simulink model "battery_dab"  (R2025a)
settings: Solver=ode1be  StartTime=0.0  StopTime=simlength  FixedStep=ts  MaxStep=ts_sim
values from neighbouring files (symbols this model uses):
  dead_time = 0    [init_model.m]
  DThs_init = 0    [init_model.m]
  fPWM_DAB = 5e3    (= 5000)    [init_model.m]
  I_FS = Iout_dc_nom * margin_factor    (= 37.5)    [init_model.m]
  Iout_dc_nom = 30    [init_model.m]
  ki_i_dab = 18    [init_model.m]
  ki_v_dab = 45    [init_model.m]
  kp_i_dab = 2    [init_model.m]
  kp_v_dab = 8    [init_model.m]
  number_of_cells = 30    [init_model.m]
  Q = 1000    [init_model.m]
  q1Kalman = ts_dab^2    (= 4e-08)    [init_model.m]
  q2Kalman = ts_dab^1    (= 0.0002)    [init_model.m]
  q3Kalman = 0    [init_model.m]
  rKalman = 1    [init_model.m]
  Tambient = 40    [init_model.m]
  tc = ts    (= 1e-06)    [init_model.m]
  ts_dab = tPWM_DAB    (= 0.0002)    [init_model.m]
  V_FS = Vout_dc_nom * margin_factor    (= 500)    [init_model.m]
  Vout_dc_nom = 400    [init_model.m]
  weigth = 0.6/6    (= 0.1)    [init_model.m]
undefined symbols (not defined in the file or in its folder): tsample
libraries: fl_lib x79, nesl_utility x61, ee_lib x13, lithium_ion_cell_lib x1, simulink x1, single_phase_transformer_lib x1
(part 1 of 4)
settings Model: SimulationMode=accelerator  Creator=LTNBDA  LastModifiedBy=dbagn
settings SolverCC: ZeroCrossControl=EnableAll  ZeroCrossAlgorithm=Adaptive  AlgebraicLoopSolver=TrustRegion  SolverResetMethod=Robust  AutoInsertRateTranBlk=on
settings DataIOCC: LimitDataPoints=on  MaxDataPoints=1  SaveFormat=Array  SignalLoggingSaveFormat=ModelDataLogs  SaveOutput=off  SignalLogging=off  DSMLogging=off  SaveTime=off  ReturnWorkspaceOutputs=off
settings OptimizationCC: ExpressionDepthLimit=2147483647.0  InitFltsAndDblsToZero=on  EfficientMapNaN2IntZero=off  LifeSpan=inf
settings DebuggingCC: SaveWithParameterizedLinksMsg=none  UnderspecifiedInitializationDetection=Classic  MergeDetectMultiDrivingBlocksExec=none  SignalResolutionControl=TryResolveAllWithWarning  SolverPrmCheckMsg=warning  MultiTaskDSMMsg=warning  MultiTaskCondExecSysMsg=none  MultiTaskRateTransMsg=warning  FcnCallInpInsideContextMsg=warning  StateNameClashWarn=warning  SFUnexpectedBacktrackingDiag=warning  SFNoUnconditionalDefaultTransitionDiag=warning  ArithmeticOperatorsInVariantConditions=warning
settings HardwareCC: ProdBitPerLong=64.0  ProdLargestAtomicFloat=None  ProdIntDivRoundTo=Undefined  ProdEndianess=Unspecified  ProdHWDeviceType=Generic->64-bit Embedded Processor (LP64)  TargetBitPerPointer=64.0  TargetBitPerSizeT=64.0  TargetBitPerPtrDiffT=64.0  TargetLongLongMode=on  TargetIntDivRoundTo=Zero  TargetEndianess=LittleEndian  TargetWordSize=64.0  TargetHWDeviceType=MATLAB Host  ProdEqTarget=off
settings ModelReferenceCC: EnableRefExpFcnMdlSchedulingChecks=on  PropagateSignalLabelsOutOfModel=off
settings SFSimCC: SimUseLocalCustomCode=off  CustomCodeUndefinedFunction=UseInterfaceOnly
settings RTWCC: RTWUseLocalCustomCode=off  GPUComputeCapability=3.5
settings CodeAppCC: MaxIdLength=128.0  StateflowObjectComments=on
settings GRTTargetCC: TargetLangStandard=C89/C90 (ANSI)  CombineOutputUpdateFcns=off  GRTInterface=on
settings ConfigComp: CovMetricSettings=dw  CovSaveCumulativeToWorkspaceVar=on  CovSaveSingleToWorkspaceVar=on  CovExternalEMLEnable=off
settings SimscapeCC: SimscapeNormalizeSystem=off

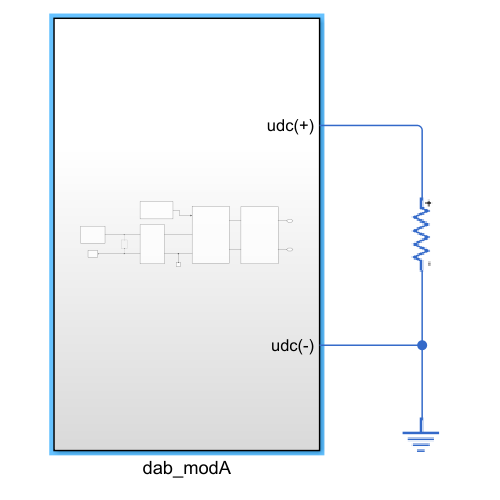
[thumbnail: Simulink's stored preview of the top-level diagram]
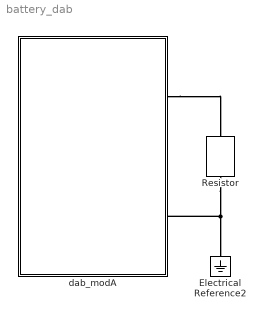
== system battery_dab ==
  Electrical Reference2 : fl_lib/Electrical/Electrical Elements/Electrical Reference
  Resistor : fl_lib/Electrical/Electrical Elements/Resistor  R=10e3 Ohm  i_specify=off  i_priority=None  i=0 A  i_nominal_specify=off  i_nominal_value=1  i_nominal_unit=A  v_specify=off  v_priority=None  v=0 V  v_nominal_specify=off  v_nominal_value=1  v_nominal_unit=V
  dab_modA : Subsystem
  connections:
  Resistor/RConn1 -- Electrical Reference2/LConn1 -- dab_modA/RConn2
  dab_modA/RConn1 -- Resistor/LConn1

== system battery_dab/dab_modA ==
  Electrical Reference : fl_lib/Electrical/Electrical Elements/Electrical Reference
  Solver Configuration : nesl_utility/Solver Configuration  PhysicalDomain=network_engine_domain  SubClassName=solver  LeftPortType=input  RightPortType=generic  Tones=[]  Harmonics=[]  SimulateNoise=off  Profile=off  UseLocalSampling=off  EnableSwitchedLinearOptims=on  FrequencyDomain=off  UseCCode=off  RelTol=0.001  AbsTol=0.001  MinStep=1e-09  ToWorkspace=off  RevertToSquareIcSolve=off  NumHomotopyIterations=100  PhasorMode=off  PhasorModeNumHarmonics=1  ConsistencySolver=NEWTON_FTOL  IndexReductionMethod=DerivativeReplacement  DoDC=on  ResidualTolerance=1e-09  ConsistencyTolSource=GLOBAL  ConsistencyAbsTol=0.001  ConsistencyRelTol=0.001  ConsistencyTolFactor=0.001  UseLocalSolver=on  LocalSolverChoice=NE_BACKWARD_EULER_ADVANCER  ResolveIndetEquations=on  FunctionEvalNumThread=1  LocalSolverSampleTime=ts  DoFixedCost=on  MaxNonlinIter=3  MaxModeIter=2  ComputeImpulses=off  ImpulseIterations=2  LinearAlgebra=auto  LinearAlgebraNumThread=0  EquationFormulation=NE_TIME_EF  DelaysMemoryBudget=1024  AutomaticFiltering=on  FilteringTimeConstant=0.001  PartitionStorageMethod=AS_NEEDED  PartitionMemoryBudget=1024  PartitionMethod=ROBUST  MultibodyUseLocalSolver=off  MultibodyLocalSolverChoice=ODE1  MultibodyLocalSolverSampleTime=0.001
  Voltage Source : ee_lib/Sources/Voltage Source  Commented=on  dc_voltage=90 V  ac_voltage=0 V  ac_shift=0 rad  ac_frequency=60 Hz  noise_mode=ee.enum.sources.noise.Disabled  PSD=0 V^2/Hz  sample_time=1e-3 s  repeatability=ee.enum.sources.repeatability.NotRepeatable  user_seed=0  auto_seed=3499211588  i_specify=off  i_priority=None  i=0 A  i_nominal_specify=off  i_nominal_value=1  i_nominal_unit=A  v_specify=off  v_priority=None  v=0 V  v_nominal_specify=off  v_nominal_value=1  v_nominal_unit=V
  battery_system : Subsystem
  dab : Subsystem
  dab_ctrl : Subsystem
  single_phase_ui_measure1 : Subsystem
  ui_measure : Subsystem
  udc(+) : PMIOPort  Side=Right
  udc(-) : PMIOPort  Port=2  Side=Right
  wires:
  dab_ctrl/1(gate_commands) -> dab/1(gate_commands)
  connections:
  dab/RConn1 -- ui_measure/LConn1
  dab/RConn2 -- ui_measure/LConn2
  udc(+)/RConn1 -- ui_measure/RConn1
  udc(-)/RConn1 -- ui_measure/RConn2
  dab/LConn2 -- single_phase_ui_measure1/RConn2 -- Electrical Reference/LConn1
  battery_system/RConn1 -- Voltage Source/LConn1 -- single_phase_ui_measure1/LConn1
  single_phase_ui_measure1/RConn1 -- dab/LConn1
  single_phase_ui_measure1/LConn2 -- Solver Configuration/RConn1 -- Voltage Source/RConn1

== system battery_dab/dab_modA/battery_system ==
  Electrical Reference1 : fl_lib/Electrical/Electrical Elements/Electrical Reference
  LithiumIonBattery : Subsystem
  Uout+ : PMIOPort  Side=Right
  connections:
  LithiumIonBattery/RConn2 -- Electrical Reference1/LConn1
  LithiumIonBattery/RConn1 -- Uout+/RConn1

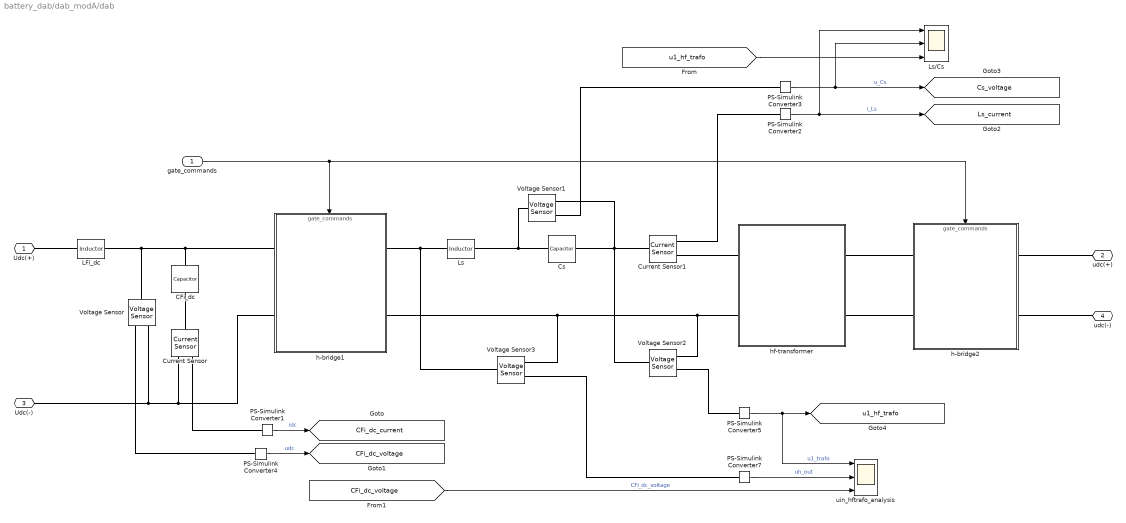
== system battery_dab/dab_modA/dab ==
  gate_commands : Inport
  CFi_dc : fl_lib/Electrical/Electrical Elements/Capacitor  c=CFi_dc F  r=RCFi_dc_internal Ohm  g=0 1/Ohm  i_specify=off  i_priority=None  i=0 A  i_nominal_specify=off  i_nominal_value=1  i_nominal_unit=A  v_specify=off  v_priority=None  v=0 V  v_nominal_specify=off  v_nominal_value=1  v_nominal_unit=V  vc_specify=off  vc_priority=High  vc=0 V  vc_nominal_specify=off  vc_nominal_value=1  vc_nominal_unit=V
  Cs : fl_lib/Electrical/Electrical Elements/Capacitor  c=Cs1 F  r=1e-6 Ohm  g=0 1/Ohm  i_specify=off  i_priority=None  i=0 A  i_nominal_specify=off  i_nominal_value=1  i_nominal_unit=A  v_specify=off  v_priority=None  v=0 V  v_nominal_specify=off  v_nominal_value=1  v_nominal_unit=V  vc_specify=off  vc_priority=High  vc=0 V  vc_nominal_specify=off  vc_nominal_value=1  vc_nominal_unit=V
  Current Sensor : fl_lib/Electrical/Electrical Sensors/Current Sensor
  Current Sensor1 : fl_lib/Electrical/Electrical Sensors/Current Sensor
  LFi_dc : fl_lib/Electrical/Electrical Elements/Inductor  l=10e-6 H  r=0 Ohm  g=1e-9 1/Ohm  i_specify=off  i_priority=None  i=0 A  i_nominal_specify=off  i_nominal_value=1  i_nominal_unit=A  v_specify=off  v_priority=None  v=0 V  v_nominal_specify=off  v_nominal_value=1  v_nominal_unit=V  i_L_specify=off  i_L_priority=High  i_L=0 A  i_L_nominal_specify=off  i_L_nominal_value=1  i_L_nominal_unit=A
  Ls : fl_lib/Electrical/Electrical Elements/Inductor  l=Ls1 H  r=0 Ohm  g=1e-9 1/Ohm  i_specify=off  i_priority=None  i=0 A  i_nominal_specify=off  i_nominal_value=1  i_nominal_unit=A  v_specify=off  v_priority=None  v=0 V  v_nominal_specify=off  v_nominal_value=1  v_nominal_unit=V  i_L_specify=off  i_L_priority=High  i_L=0 A  i_L_nominal_specify=off  i_L_nominal_value=1  i_L_nominal_unit=A
  Ls/Cs : Scope  NumInputPorts=3
      settings: SampleTime=tc  ActiveDisplayYMinimum=1.6E-10  ActiveDisplayYMaximum=3.6E-10
  PS-Simulink Converter1 : nesl_utility/PS-Simulink Converter  PhysicalDomain=network_engine_domain  SubClassName=ps_output  LeftPortType=input  RightPortType=output  PseudoPeriodic=off  Frequencies=[]  VectorFormat=1-D array  Unit=A  AffineConversion=on
  PS-Simulink Converter2 : nesl_utility/PS-Simulink Converter  PhysicalDomain=network_engine_domain  SubClassName=ps_output  LeftPortType=input  RightPortType=output  PseudoPeriodic=off  Frequencies=[]  VectorFormat=1-D array  Unit=A  AffineConversion=on
  PS-Simulink Converter{3..5,7} (4 alike) : nesl_utility/PS-Simulink Converter  PhysicalDomain=network_engine_domain  SubClassName=ps_output  LeftPortType=input  RightPortType=output  PseudoPeriodic=off  Frequencies=[]  VectorFormat=1-D array  Unit=V  AffineConversion=on
  Voltage Sensor{,1..3} (4 alike) : fl_lib/Electrical/Electrical Sensors/Voltage Sensor
  h-bridge1 : Subsystem
      settings: PortSchema="{\"entries\":[{\"content\":{\"sides\":[{\"content\":{\"connectorIds\":[\"LConn1\",\"LConn2\"]},\"type\":\"ConnectorPlacement.EquallySpacedRectSide\",\"uuid\":\"c872503a-61af-4937-bdf2-4de4f8645573\"},{\"content\":{\"connectorIds\":[\"RConn1\",\"RConn2\"],\"side\":\"RIGHT\"},\"type\":\"ConnectorPlacement.EquallySpacedRectSide\",\"uuid\":\"3b83f060-86a2-4569-84b5-d9f7c0485347\"},{\"content\":{\"connectorIds\":[\"In1\"],\"side\":\"TOP\"},\"type\":\"ConnectorPlacement.EquallySpacedRectSide\",\"uuid\":\"bf191d46-ce71-4d15-9dd0-24cc57253577\"}]},\"type\":\"ConnectorPlacement.EquallySpacedConnector\",\"uuid\":\"1b28ceee-25d0-45ae-a3c4-c2563f0d63ba\"}],\"packageUris\":[\"http://schema.mathworks.com/mf0/Connector/R2020b\"],\"version\":\"1.0\"}"
  h-bridge2 : Subsystem
      settings: PortSchema="{\"entries\":[{\"content\":{\"sides\":[{\"content\":{\"connectorIds\":[\"LConn1\",\"LConn2\"]},\"type\":\"ConnectorPlacement.EquallySpacedRectSide\",\"uuid\":\"c872503a-61af-4937-bdf2-4de4f8645573\"},{\"content\":{\"connectorIds\":[\"RConn1\",\"RConn2\"],\"side\":\"RIGHT\"},\"type\":\"ConnectorPlacement.EquallySpacedRectSide\",\"uuid\":\"3b83f060-86a2-4569-84b5-d9f7c0485347\"},{\"content\":{\"connectorIds\":[\"In1\"],\"side\":\"TOP\"},\"type\":\"ConnectorPlacement.EquallySpacedRectSide\",\"uuid\":\"bf191d46-ce71-4d15-9dd0-24cc57253577\"}]},\"type\":\"ConnectorPlacement.EquallySpacedConnector\",\"uuid\":\"1b28ceee-25d0-45ae-a3c4-c2563f0d63ba\"}],\"packageUris\":[\"http://schema.mathworks.com/mf0/Connector/R2020b\"],\"version\":\"1.0\"}"
  hf-transformer : Subsystem
  uin_hftrafo_analysis : Scope  NumInputPorts=3
      settings: SampleTime=tc  ActiveDisplayYMinimum=-95.8679  ActiveDisplayYMaximum=95.88555
  Udc(+) : PMIOPort  Side=Left
  udc(+) : PMIOPort  Port=2  Side=Right
  Udc(-) : PMIOPort  Port=3  Side=Left
  udc(-) : PMIOPort  Port=4  Side=Right
  tag scope: CFi_dc_current=global, CFi_dc_voltage=global, Cs_voltage=global, Ls_current=global, u1_hf_trafo=global
  wires:
  gate_commands/1 -> h-bridge2/1(gate_commands), h-bridge1/1(gate_commands)
  PS-Simulink Converter1/1 -> [CFi_dc_current]  "idc"
  PS-Simulink Converter4/1 -> [CFi_dc_voltage]  "udc"
  PS-Simulink Converter2/1 -> Ls/Cs/1, [Ls_current]  "i_Ls"
  PS-Simulink Converter3/1 -> Ls/Cs/2, [Cs_voltage]  "u_Cs"
  PS-Simulink Converter5/1 -> uin_hftrafo_analysis/1, [u1_hf_trafo]  "u1_trafo"
  [u1_hf_trafo] -> Ls/Cs/3
  PS-Simulink Converter7/1 -> uin_hftrafo_analysis/2  "uh_out"
  [CFi_dc_voltage] -> uin_hftrafo_analysis/3  "CFi_dc_voltage"
  connections:
  hf-transformer/LConn2 -- Voltage Sensor2/RConn2 -- Voltage Sensor3/RConn2 -- h-bridge1/LConn2
  h-bridge1/RConn1 -- CFi_dc/LConn1 -- LFi_dc/RConn1 -- Voltage Sensor/LConn1
  h-bridge1/RConn2 -- Current Sensor/RConn2 -- Udc(-)/RConn1 -- Voltage Sensor/RConn2
  LFi_dc/LConn1 -- Udc(+)/RConn1
  Current Sensor/LConn1 -- CFi_dc/RConn1
  Current Sensor/RConn1 -- PS-Simulink Converter1/LConn1
  PS-Simulink Converter4/LConn1 -- Voltage Sensor/RConn1
  h-bridge1/LConn1 -- Voltage Sensor3/LConn1 -- Ls/LConn1
  Current Sensor1/RConn2 -- hf-transformer/LConn1
  PS-Simulink Converter2/LConn1 -- Current Sensor1/RConn1
  Voltage Sensor1/RConn1 -- PS-Simulink Converter3/LConn1
  Voltage Sensor2/RConn1 -- PS-Simulink Converter5/LConn1
  Voltage Sensor1/RConn2 -- Cs/RConn1 -- Current Sensor1/LConn1 -- Voltage Sensor2/LConn1
  Ls/RConn1 -- Voltage Sensor1/LConn1 -- Cs/LConn1
  Voltage Sensor3/RConn1 -- PS-Simulink Converter7/LConn1
  hf-transformer/RConn1 -- h-bridge2/LConn1
  hf-transformer/RConn2 -- h-bridge2/LConn2
  udc(+)/RConn1 -- h-bridge2/RConn1
  udc(-)/RConn1 -- h-bridge2/RConn2

== system battery_dab/dab_modA/dab_ctrl ==
  Bus Creator : BusCreator  Inputs=8
  modulator1 : Subsystem
  references : Subsystem
  sampling_i_filter1 : Subsystem
  sampling_v_filter1 : Subsystem
  sampling_v_filter2 : Subsystem
  vi ctrl : Subsystem
  gate_commands : Outport
  wires:
  [dab_voltage_output_modA] -> sampling_v_filter1/1(in)
  [dab_current_output_modA] -> sampling_i_filter1/1(in)
  vi ctrl/1(phase_displacement) -> modulator1/1(phase_displacement)
  sampling_i_filter1/1(out_pu) -> vi ctrl/1(iout)
  sampling_v_filter1/1(out_pu) -> vi ctrl/2(vout)
  sampling_v_filter2/1(out_pu) -> vi ctrl/3(vout_ref)
  references/1(vout_ref) -> sampling_v_filter2/1(in)
  Bus Creator/1 -> gate_commands/1
  modulator1/1(gate_Q1) -> Bus Creator/1
  modulator1/2(gate_Q2) -> Bus Creator/2
  modulator1/3(gate_Q3) -> Bus Creator/3
  modulator1/4(gate_Q4) -> Bus Creator/4
  modulator1/5(gate_Q5) -> Bus Creator/5
  modulator1/6(gate_Q6) -> Bus Creator/6
  modulator1/7(gate_Q7) -> Bus Creator/7
  modulator1/8(gate_Q8) -> Bus Creator/8

== system battery_dab/dab_modA/single_phase_ui_measure1 ==
  Bus Creator : BusCreator  Inputs=2
  Current Sensor : fl_lib/Electrical/Electrical Sensors/Current Sensor
  Selector : Selector  InputPortWidth=2  IndexOptions=Index vector (dialog)  Indices=2  OutputSizes=1
  Selector1 : Selector  InputPortWidth=2  IndexOptions=Index vector (dialog)  Indices=1  OutputSizes=1
  Voltage Sensor : fl_lib/Electrical/Electrical Sensors/Voltage Sensor
  input : Scope  NumInputPorts=2
      settings: SampleTime=tc  ActiveDisplayYMinimum=-46.75689  ActiveDisplayYMaximum=366.30967  DataLoggingVariableName=ScopeData2
  iph : nesl_utility/PS-Simulink Converter  PhysicalDomain=network_engine_domain  SubClassName=ps_output  LeftPortType=input  RightPortType=output  PseudoPeriodic=off  Frequencies=[]  VectorFormat=1-D array  Unit=A  AffineConversion=off
  uph : nesl_utility/PS-Simulink Converter  PhysicalDomain=network_engine_domain  SubClassName=ps_output  LeftPortType=input  RightPortType=output  PseudoPeriodic=off  Frequencies=[]  VectorFormat=1-D array  Unit=V  AffineConversion=off
  Udc(+) : PMIOPort  Side=Left
  udc(+) : PMIOPort  Port=2  Side=Right
  Udc(-) : PMIOPort  Port=3  Side=Left
  udc(-) : PMIOPort  Port=4  Side=Right
  tag scope: current_battery=global, voltage_battery=global
  wires:
  Bus Creator/1 -> Selector/1, Selector1/1  "ui_data"
  iph/1 -> Bus Creator/1  "iph"
  uph/1 -> Bus Creator/2  "uph"
  Selector1/1 -> [current_battery], input/1  "current_battery"
  Selector/1 -> input/2, [voltage_battery]  "voltage_battery"
  connections:
  iph/LConn1 -- Current Sensor/RConn1
  Voltage Sensor/LConn1 -- Current Sensor/LConn1 -- Udc(+)/RConn1
  Current Sensor/RConn2 -- udc(+)/RConn1
  Voltage Sensor/RConn1 -- uph/LConn1
  Voltage Sensor/RConn2 -- Udc(-)/RConn1 -- udc(-)/RConn1

== system battery_dab/dab_modA/ui_measure ==
  Bus Creator : BusCreator  Inputs=2
  Current Sensor : fl_lib/Electrical/Electrical Sensors/Current Sensor
  Selector : Selector  InputPortWidth=2  IndexOptions=Index vector (dialog)  Indices=2  OutputSizes=1
  Selector1 : Selector  InputPortWidth=2  IndexOptions=Index vector (dialog)  Indices=1  OutputSizes=1
  Voltage Sensor : fl_lib/Electrical/Electrical Sensors/Voltage Sensor
  idc/udc dab modA : Scope  NumInputPorts=2
      settings: SampleTime=tc  ActiveDisplayYMinimum=4E-31  ActiveDisplayYMaximum=1.7E-30  DataLoggingVariableName=ScopeData2
  iph : nesl_utility/PS-Simulink Converter  PhysicalDomain=network_engine_domain  SubClassName=ps_output  LeftPortType=input  RightPortType=output  PseudoPeriodic=off  Frequencies=[]  VectorFormat=1-D array  Unit=A  AffineConversion=off
  uph : nesl_utility/PS-Simulink Converter  PhysicalDomain=network_engine_domain  SubClassName=ps_output  LeftPortType=input  RightPortType=output  PseudoPeriodic=off  Frequencies=[]  VectorFormat=1-D array  Unit=V  AffineConversion=off
  Udc(+) : PMIOPort  Side=Left
  udc(+) : PMIOPort  Port=2  Side=Right
  Udc(-) : PMIOPort  Port=3  Side=Left
  udc(-) : PMIOPort  Port=4  Side=Right
  tag scope: dab_current_output_modA=global, dab_voltage_output_modA=global
  wires:
  [dab_current_output_modA] -> idc/udc dab modA/1  "dab_current_output_modA"
  [dab_voltage_output_modA] -> idc/udc dab modA/2  "zvs_voltage_output_modA"
  Selector1/1 -> [dab_current_output_modA]
  Selector/1 -> [dab_voltage_output_modA]
  Bus Creator/1 -> Selector/1, Selector1/1  "ui_data"
  iph/1 -> Bus Creator/1  "iph"
  uph/1 -> Bus Creator/2  "uph"
  connections:
  iph/LConn1 -- Current Sensor/RConn1
  Voltage Sensor/LConn1 -- Current Sensor/LConn1 -- Udc(+)/RConn1
  Current Sensor/RConn2 -- udc(+)/RConn1
  Voltage Sensor/RConn1 -- uph/LConn1
  Voltage Sensor/RConn2 -- Udc(-)/RConn1 -- udc(-)/RConn1

== system battery_dab/dab_modA/battery_system/LithiumIonBattery ==
  Current Sensor : fl_lib/Electrical/Electrical Sensors/Current Sensor
  Electrical Reference1 : fl_lib/Electrical/Electrical Elements/Electrical Reference
  PS-Simulink Converter4 : nesl_utility/PS-Simulink Converter  PhysicalDomain=network_engine_domain  SubClassName=ps_output  LeftPortType=input  RightPortType=output  PseudoPeriodic=off  Frequencies=[]  VectorFormat=1-D array  Unit=1  AffineConversion=off
  PS-Simulink Converter5 : nesl_utility/PS-Simulink Converter  PhysicalDomain=network_engine_domain  SubClassName=ps_output  LeftPortType=input  RightPortType=output  PseudoPeriodic=off  Frequencies=[]  VectorFormat=1-D array  Unit=V  AffineConversion=on
  SOC_estimator : Subsystem
  To Workspace1 : ToWorkspace  VariableName=idc_battery_sim  SampleTime=tc
      settings: MaxDataPoints=Nc
  To Workspace2 : ToWorkspace  VariableName=udc_battery_sim  SampleTime=tc
      settings: MaxDataPoints=Nc
  Unit Delay5 : UnitDelay  SampleTime=ts_dab  HasFrameUpgradeWarning=on
  Voltage Sensor : fl_lib/Electrical/Electrical Sensors/Voltage Sensor
  ibat/vdc : Scope  NumInputPorts=2
      settings: SampleTime=tc  ActiveDisplayYMinimum=102.29193  ActiveDisplayYMaximum=106.82602  DataLoggingVariableName=ScopeData6
  lithium ion cell analytical ocv : Subsystem
  Uout+ : PMIOPort  Side=Right
  Uout- : PMIOPort  Port=2  Side=Right
  wires:
  PS-Simulink Converter5/1 -> Unit Delay5/1
  PS-Simulink Converter4/1 -> To Workspace1/1, ibat/vdc/1  "i batt"
  Unit Delay5/1 -> To Workspace2/1, [vdc]
  [vdc] -> ibat/vdc/2  "vdc"
  connections:
  Current Sensor/RConn1 -- PS-Simulink Converter4/LConn1
  Uout+/RConn1 -- Current Sensor/RConn2 -- Voltage Sensor/LConn1
  Voltage Sensor/RConn1 -- PS-Simulink Converter5/LConn1
  Voltage Sensor/RConn2 -- Electrical Reference1/LConn1 -- lithium ion cell analytical ocv/RConn2 -- Uout-/RConn1
  lithium ion cell analytical ocv/RConn1 -- Current Sensor/LConn1

== system battery_dab/dab_modA/dab/h-bridge1 ==
  gate_commands : Inport
  Current Sensor : fl_lib/Electrical/Electrical Sensors/Current Sensor
  PS-Simulink Converter1 : nesl_utility/PS-Simulink Converter  PhysicalDomain=network_engine_domain  SubClassName=ps_output  LeftPortType=input  RightPortType=output  PseudoPeriodic=off  Frequencies=[]  VectorFormat=1-D array  Unit=A  AffineConversion=on
  h-bridge_thermal : Subsystem  Commented=on
  h-ideal : Subsystem  Commented=on
  h-mosfet : Subsystem
  uac_1(+) : PMIOPort  Side=Left
  uac_1(-) : PMIOPort  Port=2  Side=Left
  Udc(+) : PMIOPort  Port=3  Side=Right
  Udc(-) : PMIOPort  Port=4  Side=Right
  tag scope: dc_bus_terminal_current_inverter=global
  wires:
  gate_commands/1 -> h-mosfet/1(gate_commands)
  PS-Simulink Converter1/1 -> [dc_bus_terminal_current_inverter]  "idc"
  connections:
  h-mosfet/LConn1 -- uac_1(+)/RConn1
  h-mosfet/LConn2 -- uac_1(-)/RConn1
  h-mosfet/RConn2 -- Udc(-)/RConn1
  Current Sensor/LConn1 -- Udc(+)/RConn1
  h-mosfet/RConn1 -- Current Sensor/RConn2
  PS-Simulink Converter1/LConn1 -- Current Sensor/RConn1

== system battery_dab/dab_modA/dab/h-bridge2 ==
  gate_commands : Inport
  CFu_dc : fl_lib/Electrical/Electrical Elements/Capacitor  c=CFu_dc F  r=RCFu_dc_internal Ohm  g=0 1/Ohm  i_specify=off  i_priority=None  i=0 A  i_nominal_specify=off  i_nominal_value=1  i_nominal_unit=A  v_specify=off  v_priority=None  v=0 V  v_nominal_specify=off  v_nominal_value=1  v_nominal_unit=V  vc_specify=off  vc_priority=High  vc=0 V  vc_nominal_specify=off  vc_nominal_value=1  vc_nominal_unit=V
  Current Sensor : fl_lib/Electrical/Electrical Sensors/Current Sensor
  Current Sensor2 : fl_lib/Electrical/Electrical Sensors/Current Sensor
  PS-Simulink Converter1 : nesl_utility/PS-Simulink Converter  PhysicalDomain=network_engine_domain  SubClassName=ps_output  LeftPortType=input  RightPortType=output  PseudoPeriodic=off  Frequencies=[]  VectorFormat=1-D array  Unit=A  AffineConversion=on
  PS-Simulink Converter6 : nesl_utility/PS-Simulink Converter  PhysicalDomain=network_engine_domain  SubClassName=ps_output  LeftPortType=input  RightPortType=output  PseudoPeriodic=off  Frequencies=[]  VectorFormat=1-D array  Unit=A  AffineConversion=on
  PS-Simulink Converter8 : nesl_utility/PS-Simulink Converter  PhysicalDomain=network_engine_domain  SubClassName=ps_output  LeftPortType=input  RightPortType=output  PseudoPeriodic=off  Frequencies=[]  VectorFormat=1-D array  Unit=V  AffineConversion=on
  Voltage Sensor4 : fl_lib/Electrical/Electrical Sensors/Voltage Sensor
  h-mosfet : Subsystem
  uac_1(+) : PMIOPort  Side=Left
  uac_1(-) : PMIOPort  Port=2  Side=Left
  udc(+) : PMIOPort  Port=3  Side=Right
  udc(-) : PMIOPort  Port=4  Side=Right
  tag scope: CFu_dc_current=global, CFu_dc_voltage=global
  wires:
  gate_commands/1 -> h-mosfet/1(gate_commands)
  PS-Simulink Converter6/1 -> [CFu_dc_current]  "i_Ls"
  PS-Simulink Converter8/1 -> [CFu_dc_voltage]  "CFu_dc_voltage"
  connections:
  h-mosfet/RConn1 -- Current Sensor/LConn1 -- CFu_dc/LConn1
  Voltage Sensor4/LConn1 -- udc(+)/RConn1 -- Current Sensor/RConn2
  h-mosfet/RConn2 -- Current Sensor2/RConn2 -- udc(-)/RConn1 -- Voltage Sensor4/RConn2
  h-mosfet/LConn2 -- uac_1(-)/RConn1
  h-mosfet/LConn1 -- uac_1(+)/RConn1
  Voltage Sensor4/RConn1 -- PS-Simulink Converter8/LConn1
  PS-Simulink Converter6/LConn1 -- Current Sensor2/RConn1
  CFu_dc/RConn1 -- Current Sensor2/LConn1
  Current Sensor/RConn1 -- PS-Simulink Converter1/LConn1

== system battery_dab/dab_modA/dab/hf-transformer ==
  Current Sensor1 : fl_lib/Electrical/Electrical Sensors/Current Sensor
  PS-Simulink Converter2 : nesl_utility/PS-Simulink Converter  PhysicalDomain=network_engine_domain  SubClassName=ps_output  LeftPortType=input  RightPortType=output  PseudoPeriodic=off  Frequencies=[]  VectorFormat=1-D array  Unit=A  AffineConversion=on
  hf_trafo_center_tap_ss : Subsystem
  uac_1(+) : PMIOPort  Side=Left
  uac_2(+) : PMIOPort  Port=2  Side=Right
  uac_1(-) : PMIOPort  Port=3  Side=Left
  uac_2(-) : PMIOPort  Port=4  Side=Right
  connections:
  Current Sensor1/RConn2 -- uac_2(+)/RConn1
  PS-Simulink Converter2/LConn1 -- Current Sensor1/RConn1
  hf_trafo_center_tap_ss/LConn1 -- uac_1(+)/RConn1
  hf_trafo_center_tap_ss/RConn1 -- Current Sensor1/LConn1
  hf_trafo_center_tap_ss/LConn2 -- uac_1(-)/RConn1
  hf_trafo_center_tap_ss/RConn2 -- uac_2(-)/RConn1

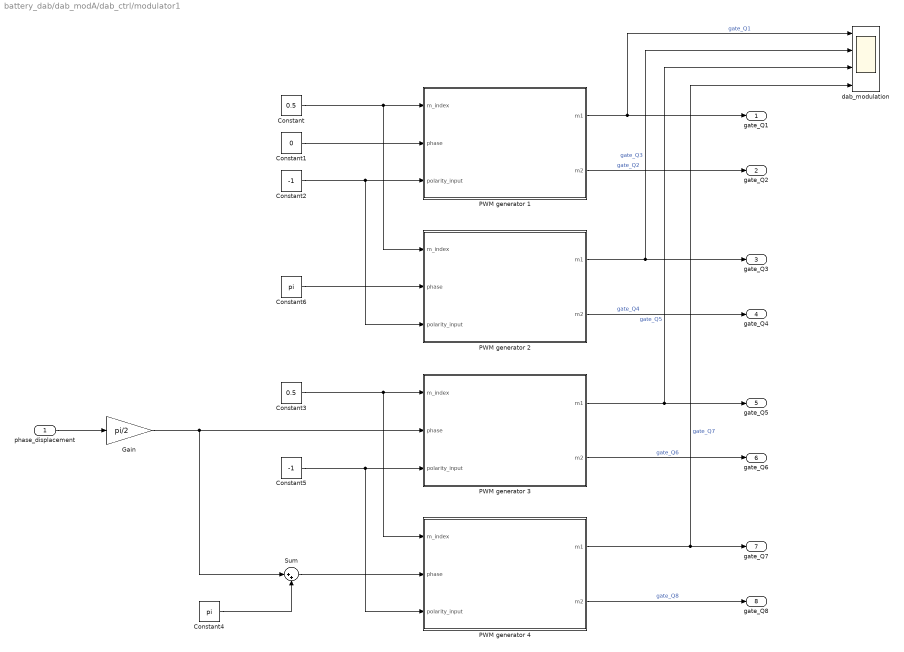
== system battery_dab/dab_modA/dab_ctrl/modulator1 ==
  phase_displacement : Inport
  Constant : Constant  Value=0.5
  Constant1 : Constant  Value=0
  Constant2 : Constant  Value=-1
  Constant3 : Constant  Value=0.5
  Constant4 : Constant  Value=pi
  Constant5 : Constant  Value=-1
  Constant6 : Constant  Value=pi
  Gain : Gain  Gain=pi/2  OutDataTypeStr=double
  PWM generator 1 : Subsystem  mask{f=fPWM_DAB, m_up=1, m_low=0, dead_time=dead_time, pos_cmd_gate=15, neg_cmd_gate=-10, polarity=1}
      mask prompts: f "Frequency (Hz)"; m_up "Max Input Modulation Value"; m_low "Min Input Modulation Value"; dead_time "Dead Time (s)"; pos_cmd_gate "Positive Gate Voltage (V)"; neg_cmd_gate "Negative Gate Voltage (V)"; polarity "Polarity (pu)"
  PWM generator 2 : Subsystem  mask{f=fPWM_DAB, m_up=1, m_low=0, dead_time=dead_time, pos_cmd_gate=15, neg_cmd_gate=-10, polarity=1}
      mask prompts: f "Frequency (Hz)"; m_up "Max Input Modulation Value"; m_low "Min Input Modulation Value"; dead_time "Dead Time (s)"; pos_cmd_gate "Positive Gate Voltage (V)"; neg_cmd_gate "Negative Gate Voltage (V)"; polarity "Polarity (pu)"
  PWM generator 3 : Subsystem  mask{f=fPWM_DAB, m_up=1, m_low=0, dead_time=dead_time, pos_cmd_gate=15, neg_cmd_gate=-10, polarity=1}
      mask prompts: f "Frequency (Hz)"; m_up "Max Input Modulation Value"; m_low "Min Input Modulation Value"; dead_time "Dead Time (s)"; pos_cmd_gate "Positive Gate Voltage (V)"; neg_cmd_gate "Negative Gate Voltage (V)"; polarity "Polarity (pu)"
  PWM generator 4 : Subsystem  mask{f=fPWM_DAB, m_up=1, m_low=0, dead_time=dead_time, pos_cmd_gate=15, neg_cmd_gate=-10, polarity=1}
      mask prompts: f "Frequency (Hz)"; m_up "Max Input Modulation Value"; m_low "Min Input Modulation Value"; dead_time "Dead Time (s)"; pos_cmd_gate "Positive Gate Voltage (V)"; neg_cmd_gate "Negative Gate Voltage (V)"; polarity "Polarity (pu)"
  Sum : Sum  Inputs=|++
  dab_modulation : Scope  NumInputPorts=4
      settings: SampleTime=tc  ActiveDisplayYMinimum=-13.125  ActiveDisplayYMaximum=18.125
  gate_Q1 : Outport
  gate_Q2 : Outport  Port=2
  gate_Q3 : Outport  Port=3
  gate_Q4 : Outport  Port=4
  gate_Q5 : Outport  Port=5
  gate_Q6 : Outport  Port=6
  gate_Q7 : Outport  Port=7
  gate_Q8 : Outport  Port=8
  wires:
  PWM generator 2/2(m2) -> gate_Q4/1  "gate_Q4"
  PWM generator 2/1(m1) -> dab_modulation/2, gate_Q3/1  "gate_Q3"
  PWM generator 1/2(m2) -> gate_Q2/1  "gate_Q2"
  PWM generator 1/1(m1) -> gate_Q1/1, dab_modulation/1  "gate_Q1"
  phase_displacement/1 -> Gain/1
  Constant/1 -> PWM generator 2/1(m_index), PWM generator 1/1(m_index)
  Constant1/1 -> PWM generator 1/2(phase)
  Constant2/1 -> PWM generator 2/3(polarity_input), PWM generator 1/3(polarity_input)
  Constant5/1 -> PWM generator 3/3(polarity_input), PWM generator 4/3(polarity_input)
  Gain/1 -> Sum/1, PWM generator 3/2(phase)
  Constant3/1 -> PWM generator 3/1(m_index), PWM generator 4/1(m_index)
  Sum/1 -> PWM generator 4/2(phase)
  PWM generator 3/1(m1) -> gate_Q5/1, dab_modulation/3  "gate_Q5"
  PWM generator 3/2(m2) -> gate_Q6/1  "gate_Q6"
  PWM generator 4/1(m1) -> dab_modulation/4, gate_Q7/1  "gate_Q7"
  PWM generator 4/2(m2) -> gate_Q8/1  "gate_Q8"
  Constant6/1 -> PWM generator 2/2(phase)
  Constant4/1 -> Sum/2

== system battery_dab/dab_modA/dab_ctrl/references ==
  voltage_reference : Subsystem
  vout_ref : Outport
  wires:
  voltage_reference/1(vout_ref) -> vout_ref/1

== system battery_dab/dab_modA/dab_ctrl/sampling_i_filter1 ==
  in : Inport
  1/Ti3 : Gain  Gain=1/I_FS  OutDataTypeStr=double  SaturateOnIntegerOverflow=on  ParamDataTypeStr=Inherit: Same as input
  Saturation : Saturate  UpperLimit=1  LowerLimit=0  OutDataTypeStr=double
  Zero-Order Hold2 : ZeroOrderHold  SampleTime=ts_dab
  out_pu : Outport
  wires:
  in/1 -> 1/Ti3/1
  1/Ti3/1 -> Saturation/1
  Saturation/1 -> Zero-Order Hold2/1
  Zero-Order Hold2/1 -> out_pu/1

== system battery_dab/dab_modA/dab_ctrl/sampling_v_filter1 ==
  in : Inport
  1/Ti3 : Gain  Gain=1/V_FS  OutDataTypeStr=double  SaturateOnIntegerOverflow=on  ParamDataTypeStr=Inherit: Same as input
  Saturation : Saturate  UpperLimit=1  LowerLimit=0  OutDataTypeStr=double
  Zero-Order Hold2 : ZeroOrderHold  SampleTime=ts_dab
  out_pu : Outport
  wires:
  Zero-Order Hold2/1 -> out_pu/1
  1/Ti3/1 -> Saturation/1
  in/1 -> 1/Ti3/1
  Saturation/1 -> Zero-Order Hold2/1

== system battery_dab/dab_modA/dab_ctrl/sampling_v_filter2 ==
  in : Inport
  1/Ti3 : Gain  Gain=1/V_FS  OutDataTypeStr=double  SaturateOnIntegerOverflow=on  ParamDataTypeStr=Inherit: Same as input
  Saturation : Saturate  UpperLimit=1  LowerLimit=0  OutDataTypeStr=double
  Zero-Order Hold2 : ZeroOrderHold  SampleTime=ts_dab
  out_pu : Outport
  wires:
  Saturation/1 -> Zero-Order Hold2/1
  in/1 -> 1/Ti3/1
  1/Ti3/1 -> Saturation/1
  Zero-Order Hold2/1 -> out_pu/1

== system battery_dab/dab_modA/dab_ctrl/vi ctrl ==
  iout : Inport
  vout : Inport  Port=2
  vout_ref : Inport  Port=3
  Constant : Constant  Value=Iout_dc_nom
  Iout Ctrl : Subsystem
  Min : MinMax  Inputs=2
  To Workspace1 : ToWorkspace  VariableName=phase_ctrl_out_modA_sim  SampleTime=ts_dab
      settings: MaxDataPoints=Ns_dab
  To Workspace2 : ToWorkspace  VariableName=pid_ctrlv_out_modA_sim  SampleTime=ts_dab
      settings: MaxDataPoints=Ns_dab
  To Workspace3 : ToWorkspace  VariableName=pid_ctrli_out_modA_sim  SampleTime=ts_dab
      settings: MaxDataPoints=Ns_dab
  Unit Delay2 : UnitDelay  SampleTime=ts_dab  HasFrameUpgradeWarning=on
  Vout Ctrl : Subsystem
  zvs_ctrl : Scope  NumInputPorts=2
      settings: SampleTime=tc  ActiveDisplayYMinimum=-1.16562  ActiveDisplayYMaximum=0.4906
  phase_displacement : Outport
  wires:
  Unit Delay2/1 -> phase_displacement/1, To Workspace1/1
  iout/1 -> Iout Ctrl/2(iout)
  vout_ref/1 -> Vout Ctrl/1(vout_ref)
  vout/1 -> Vout Ctrl/2(vout)
  Vout Ctrl/1(ctrlv_out) -> zvs_ctrl/1, Unit Delay2/1, To Workspace2/1  "u_ctrl_out"
  Constant/1 -> Iout Ctrl/1(iout_ref)
  Iout Ctrl/1(ctrli_out) -> zvs_ctrl/2, To Workspace3/1, Min/2  "i_ctrl_out"

== system battery_dab/dab_modA/battery_system/LithiumIonBattery/SOC_estimator ==
  Kalman_observer : Subsystem
  SOC*/SOC : Scope  Commented=on  NumInputPorts=2
      settings: SampleTime=tsample  ActiveDisplayYMinimum=-0.16149  ActiveDisplayYMaximum=0.90685
  Selector1 : Selector  InputPortWidth=3  IndexOptions=Index vector (dialog)  Indices=3  OutputSizes=1
  h_hat/h : Scope  Commented=on  NumInputPorts=2
      settings: SampleTime=tsample  ActiveDisplayYMinimum=-0.13002  ActiveDisplayYMaximum=0.15534  DataLoggingVariableName=ScopeData2
  i_out/v_out : Scope  Commented=on  NumInputPorts=2
      settings: SampleTime=tsample  ActiveDisplayYMinimum=-467.64425  ActiveDisplayYMaximum=280.87629  DataLoggingVariableName=ScopeData3
  soc/iout : Scope  Commented=on  NumInputPorts=2
      settings: SampleTime=tsample  ActiveDisplayYMinimum=0.19925  ActiveDisplayYMaximum=0.20008  DataLoggingVariableName=ScopeData4
  wires:
  Kalman_observer/2(SOC) -> SOC*/SOC/2
  Kalman_observer/1(x(k+1|k)) -> Selector1/1
  [im] -> i_out/v_out/1  "im+noise"
  [h] -> h_hat/h/2
  [SOC] -> soc/iout/1, SOC*/SOC/1
  Selector1/1 -> h_hat/h/1  "h_hat(z)"
  [vout] -> Kalman_observer/1(vout(k)), i_out/v_out/2
  [icell] -> soc/iout/2

== system battery_dab/dab_modA/battery_system/LithiumIonBattery/lithium ion cell analytical ocv ==
  Current Sensor : fl_lib/Electrical/Electrical Sensors/Current Sensor
  Electrical Reference : fl_lib/Electrical/Electrical Elements/Electrical Reference
  PS Constant : fl_lib/Physical Signals/Sources/PS Constant  constant=298.15 K
  PS-Simulink Converter{,1..4} (5 alike) : nesl_utility/PS-Simulink Converter  PhysicalDomain=network_engine_domain  SubClassName=ps_output  LeftPortType=input  RightPortType=output  PseudoPeriodic=off  Frequencies=[]  VectorFormat=1-D array  Unit=inherit  AffineConversion=off
  Voltage Sensor : fl_lib/Electrical/Electrical Sensors/Voltage Sensor
  lithium-ion battery with analytical OCV : lithium_ion_cell_lib/lithium-ion Cell with analytical OCV  Qcell=Q hr*A  N=number_of_cells  E_1=E1 V  E0=E0 V  E1=E1 V  E2=E2 V  E3=E3 V  Elog=Elog V  R0=R0 Ohm  R1=R1 Ohm  C1=C1 F  M=M V  alpha=alpha  u_specify=off  u_priority=High  u=Vdc V  u_nominal_specify=off  u_nominal_unit=V  u_nominal_value=1  u_ocv_specify=off  u_ocv_priority=High  u_ocv=Vdc V  u_ocv_nominal_specify=off  u_ocv_nominal_unit=V  u_ocv_nominal_value=1  icell_specify=off  icell_priority=None  icell=0 A  icell_nominal_specify=off  icell_nominal_unit=A  icell_nominal_value=1  i_r1_specify=off  i_r1_priority=None  i_r1=0 A  i_r1_nominal_specify=off  i_r1_nominal_unit=A  i_r1_nominal_value=1  z_specify=on  z_priority=High  z=soc_init  z_nominal_specify=off  z_nominal_unit=1  z_nominal_value=1  h_specify=off  h_priority=High  h=0  h_nominal_specify=off  h_nominal_unit=1  h_nominal_value=1
      settings: InternalSimscapePortConfiguration="{\"Bottom\":[],\"Left\":[{\"id\":\"T\",\"label\":\"T\",\"type\":\"input\"}],\"Right\":[{\"id\":\"u_p\",\"label\":\"u+\",\"type\":\"foundation.electrical.electrical\"},{\"id\":\"u_n\",\"label\":\"u-\",\"type\":\"foundation.electrical.electrical\"},{\"id\":\"z_out\",\"label\":\"SOC\",\"type\":\"output\"},{\"id\":\"i_r1_out\",\"label\":\"i_r1\",\"type\":\"output\"},{\"id\":\"h_out\",\"label\":\"hysteresis\",\"type\":\"output\"}],\"Top\":[]}"
  white_noise : Subsystem
  U+ : PMIOPort  Side=Right
  U- : PMIOPort  Port=2  Side=Right
  tag scope: SOC=global, h=global, icell=global, im=global, vout=global
  wires:
  PS-Simulink Converter/1 -> [vout]  "vout(k)"
  PS-Simulink Converter1/1 -> white_noise/1(in)  "i(k)"
  white_noise/1(out) -> [im]
  PS-Simulink Converter4/1 -> [h]  "h(t)"
  PS-Simulink Converter2/1 -> [icell]  "icell"
  PS-Simulink Converter3/1 -> [SOC]  "SOC*"
  connections:
  lithium-ion battery with analytical OCV/LConn1 -- PS Constant/RConn1
  PS-Simulink Converter/LConn1 -- Voltage Sensor/RConn1
  Current Sensor/RConn2 -- Voltage Sensor/LConn1 -- U+/RConn1
  Electrical Reference/LConn1 -- Voltage Sensor/RConn2 -- U-/RConn1 -- lithium-ion battery with analytical OCV/RConn2
  Current Sensor/RConn1 -- PS-Simulink Converter1/LConn1
  lithium-ion battery with analytical OCV/RConn1 -- Current Sensor/LConn1
  lithium-ion battery with analytical OCV/RConn3 -- PS-Simulink Converter3/LConn1
  lithium-ion battery with analytical OCV/RConn4 -- PS-Simulink Converter2/LConn1
  lithium-ion battery with analytical OCV/RConn5 -- PS-Simulink Converter4/LConn1

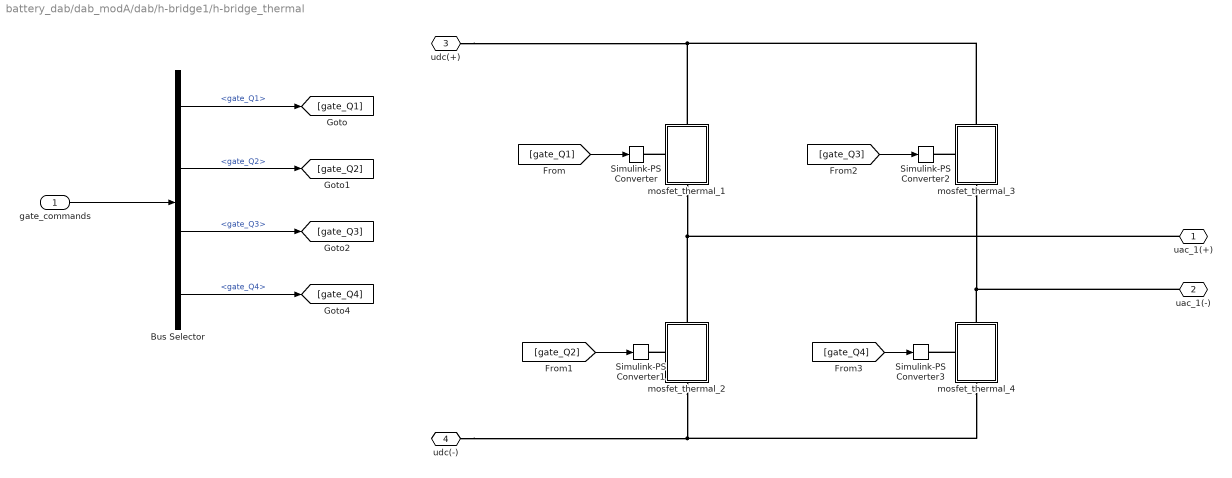
== system battery_dab/dab_modA/dab/h-bridge1/h-bridge_thermal ==
  gate_commands : Inport
  Bus Selector : BusSelector  OutputSignals=gate_Q1,gate_Q2,gate_Q3,gate_Q4
  Simulink-PS Converter{,1..3} (4 alike) : nesl_utility/Simulink-PS Converter  PhysicalDomain=network_engine_domain  SubClassName=ps_input  LeftPortType=input  RightPortType=output  PseudoPeriodic=off  Frequencies=[]  NoiseDistribution=none  NoiseParameters=[]  Unit=V  AffineConversion=off  FilteringAndDerivatives=provide  SimscapeFilterOrder=1  InputFilterTimeConstant=0.001  UdotUserProvided=0
  mosfet_thermal_1 : Subsystem
      settings: PortSchema="{\"entries\":[{\"content\":{\"sides\":[{\"content\":{\"connectorIds\":[\"LConn1\"]},\"type\":\"ConnectorPlacement.EquallySpacedRectSide\",\"uuid\":\"9277da8d-d460-43e6-8478-dd662f15d226\"},{\"content\":{\"connectorIds\":[],\"side\":\"RIGHT\"},\"type\":\"ConnectorPlacement.EquallySpacedRectSide\",\"uuid\":\"a7ece396-f1d9-4f4f-a05b-db1fc65d6e1d\"},{\"content\":{\"connectorIds\":[\"LConn2\"],\"side\":\"TOP\"},\"type\":\"ConnectorPlacement.EquallySpacedRectSide\",\"uuid\":\"fdd70777-e9cf-4317-afb6-cae87f75d5b0\"},{\"content\":{\"connectorIds\":[\"RConn1\"],\"side\":\"BOTTOM\"},\"type\":\"ConnectorPlacement.EquallySpacedRectSide\",\"uuid\":\"2353ed68-b1a1-4775-9ca9-31e268d5443b\"}]},\"type\":\"ConnectorPlacement.EquallySpacedConnector\",\"uuid\":\"d5479f4c-4e65-4791-adcb-73df11f88590\"}],\"packageUris\":[\"http://schema.mathworks.com/mf0/Connector/R2020b\"],\"version\":\"1.0\"}"
  mosfet_thermal_2 : Subsystem
      settings: PortSchema="{\"entries\":[{\"content\":{\"sides\":[{\"content\":{\"connectorIds\":[\"LConn1\"]},\"type\":\"ConnectorPlacement.EquallySpacedRectSide\",\"uuid\":\"9277da8d-d460-43e6-8478-dd662f15d226\"},{\"content\":{\"connectorIds\":[],\"side\":\"RIGHT\"},\"type\":\"ConnectorPlacement.EquallySpacedRectSide\",\"uuid\":\"a7ece396-f1d9-4f4f-a05b-db1fc65d6e1d\"},{\"content\":{\"connectorIds\":[\"LConn2\"],\"side\":\"TOP\"},\"type\":\"ConnectorPlacement.EquallySpacedRectSide\",\"uuid\":\"fdd70777-e9cf-4317-afb6-cae87f75d5b0\"},{\"content\":{\"connectorIds\":[\"RConn1\"],\"side\":\"BOTTOM\"},\"type\":\"ConnectorPlacement.EquallySpacedRectSide\",\"uuid\":\"2353ed68-b1a1-4775-9ca9-31e268d5443b\"}]},\"type\":\"ConnectorPlacement.EquallySpacedConnector\",\"uuid\":\"d5479f4c-4e65-4791-adcb-73df11f88590\"}],\"packageUris\":[\"http://schema.mathworks.com/mf0/Connector/R2020b\"],\"version\":\"1.0\"}"
  mosfet_thermal_3 : Subsystem
      settings: PortSchema="{\"entries\":[{\"content\":{\"sides\":[{\"content\":{\"connectorIds\":[\"LConn1\"]},\"type\":\"ConnectorPlacement.EquallySpacedRectSide\",\"uuid\":\"9277da8d-d460-43e6-8478-dd662f15d226\"},{\"content\":{\"connectorIds\":[],\"side\":\"RIGHT\"},\"type\":\"ConnectorPlacement.EquallySpacedRectSide\",\"uuid\":\"a7ece396-f1d9-4f4f-a05b-db1fc65d6e1d\"},{\"content\":{\"connectorIds\":[\"LConn2\"],\"side\":\"TOP\"},\"type\":\"ConnectorPlacement.EquallySpacedRectSide\",\"uuid\":\"fdd70777-e9cf-4317-afb6-cae87f75d5b0\"},{\"content\":{\"connectorIds\":[\"RConn1\"],\"side\":\"BOTTOM\"},\"type\":\"ConnectorPlacement.EquallySpacedRectSide\",\"uuid\":\"2353ed68-b1a1-4775-9ca9-31e268d5443b\"}]},\"type\":\"ConnectorPlacement.EquallySpacedConnector\",\"uuid\":\"d5479f4c-4e65-4791-adcb-73df11f88590\"}],\"packageUris\":[\"http://schema.mathworks.com/mf0/Connector/R2020b\"],\"version\":\"1.0\"}"
  mosfet_thermal_4 : Subsystem
      settings: PortSchema="{\"entries\":[{\"content\":{\"sides\":[{\"content\":{\"connectorIds\":[\"LConn1\"]},\"type\":\"ConnectorPlacement.EquallySpacedRectSide\",\"uuid\":\"9277da8d-d460-43e6-8478-dd662f15d226\"},{\"content\":{\"connectorIds\":[],\"side\":\"RIGHT\"},\"type\":\"ConnectorPlacement.EquallySpacedRectSide\",\"uuid\":\"a7ece396-f1d9-4f4f-a05b-db1fc65d6e1d\"},{\"content\":{\"connectorIds\":[\"LConn2\"],\"side\":\"TOP\"},\"type\":\"ConnectorPlacement.EquallySpacedRectSide\",\"uuid\":\"fdd70777-e9cf-4317-afb6-cae87f75d5b0\"},{\"content\":{\"connectorIds\":[\"RConn1\"],\"side\":\"BOTTOM\"},\"type\":\"ConnectorPlacement.EquallySpacedRectSide\",\"uuid\":\"2353ed68-b1a1-4775-9ca9-31e268d5443b\"}]},\"type\":\"ConnectorPlacement.EquallySpacedConnector\",\"uuid\":\"d5479f4c-4e65-4791-adcb-73df11f88590\"}],\"packageUris\":[\"http://schema.mathworks.com/mf0/Connector/R2020b\"],\"version\":\"1.0\"}"
  uac_1(+) : PMIOPort  Side=Left
  uac_1(-) : PMIOPort  Port=2  Side=Left
  udc(+) : PMIOPort  Port=3  Side=Right
  udc(-) : PMIOPort  Port=4  Side=Right
  wires:
  Bus Selector/4 -> [gate_Q4]  "<gate_Q4>"
  Bus Selector/3 -> [gate_Q3]  "<gate_Q3>"
  Bus Selector/2 -> [gate_Q2]  "<gate_Q2>"
  Bus Selector/1 -> [gate_Q1]  "<gate_Q1>"
  gate_commands/1 -> Bus Selector/1
  [gate_Q4] -> Simulink-PS Converter3/1
  [gate_Q3] -> Simulink-PS Converter2/1
  [gate_Q2] -> Simulink-PS Converter1/1
  [gate_Q1] -> Simulink-PS Converter/1
  connections:
  udc(+)/RConn1 -- mosfet_thermal_3/LConn2 -- mosfet_thermal_1/LConn2
  uac_1(-)/RConn1 -- mosfet_thermal_4/LConn2 -- mosfet_thermal_3/RConn1
  uac_1(+)/RConn1 -- mosfet_thermal_2/LConn2 -- mosfet_thermal_1/RConn1
  mosfet_thermal_4/LConn1 -- Simulink-PS Converter3/RConn1
  mosfet_thermal_3/LConn1 -- Simulink-PS Converter2/RConn1
  mosfet_thermal_2/LConn1 -- Simulink-PS Converter1/RConn1
  mosfet_thermal_1/LConn1 -- Simulink-PS Converter/RConn1
  udc(-)/RConn1 -- mosfet_thermal_4/RConn1 -- mosfet_thermal_2/RConn1

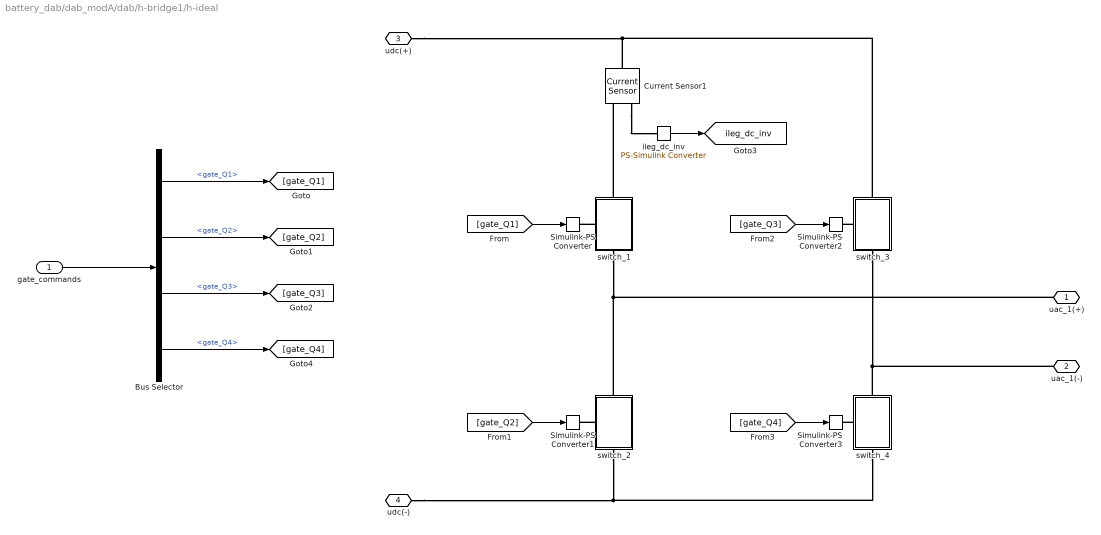
== system battery_dab/dab_modA/dab/h-bridge1/h-ideal ==
  gate_commands : Inport
  Bus Selector : BusSelector  OutputSignals=gate_Q1,gate_Q2,gate_Q3,gate_Q4
  Current Sensor1 : fl_lib/Electrical/Electrical Sensors/Current Sensor
  Simulink-PS Converter{,1..3} (4 alike) : nesl_utility/Simulink-PS Converter  PhysicalDomain=network_engine_domain  SubClassName=ps_input  LeftPortType=input  RightPortType=output  PseudoPeriodic=off  Frequencies=[]  NoiseDistribution=none  NoiseParameters=[]  Unit=1  AffineConversion=on  FilteringAndDerivatives=provide  SimscapeFilterOrder=1  InputFilterTimeConstant=0.001  UdotUserProvided=0
  ileg_dc_inv : nesl_utility/PS-Simulink Converter  PhysicalDomain=network_engine_domain  SubClassName=ps_output  LeftPortType=input  RightPortType=output  PseudoPeriodic=off  Frequencies=[]  VectorFormat=1-D array  Unit=A  AffineConversion=on
  switch_1 : Subsystem
      settings: PortSchema="{\"entries\":[{\"content\":{\"sides\":[{\"content\":{\"connectorIds\":[\"LConn1\"]},\"type\":\"ConnectorPlacement.EquallySpacedRectSide\",\"uuid\":\"9277da8d-d460-43e6-8478-dd662f15d226\"},{\"content\":{\"connectorIds\":[],\"side\":\"RIGHT\"},\"type\":\"ConnectorPlacement.EquallySpacedRectSide\",\"uuid\":\"a7ece396-f1d9-4f4f-a05b-db1fc65d6e1d\"},{\"content\":{\"connectorIds\":[\"LConn2\"],\"side\":\"TOP\"},\"type\":\"ConnectorPlacement.EquallySpacedRectSide\",\"uuid\":\"fdd70777-e9cf-4317-afb6-cae87f75d5b0\"},{\"content\":{\"connectorIds\":[\"RConn1\"],\"side\":\"BOTTOM\"},\"type\":\"ConnectorPlacement.EquallySpacedRectSide\",\"uuid\":\"2353ed68-b1a1-4775-9ca9-31e268d5443b\"}]},\"type\":\"ConnectorPlacement.EquallySpacedConnector\",\"uuid\":\"d5479f4c-4e65-4791-adcb-73df11f88590\"}],\"packageUris\":[\"http://schema.mathworks.com/mf0/Connector/R2020b\"],\"version\":\"1.0\"}"
  switch_2 : Subsystem
      settings: PortSchema="{\"entries\":[{\"content\":{\"sides\":[{\"content\":{\"connectorIds\":[\"LConn1\"]},\"type\":\"ConnectorPlacement.EquallySpacedRectSide\",\"uuid\":\"9277da8d-d460-43e6-8478-dd662f15d226\"},{\"content\":{\"connectorIds\":[],\"side\":\"RIGHT\"},\"type\":\"ConnectorPlacement.EquallySpacedRectSide\",\"uuid\":\"a7ece396-f1d9-4f4f-a05b-db1fc65d6e1d\"},{\"content\":{\"connectorIds\":[\"LConn2\"],\"side\":\"TOP\"},\"type\":\"ConnectorPlacement.EquallySpacedRectSide\",\"uuid\":\"fdd70777-e9cf-4317-afb6-cae87f75d5b0\"},{\"content\":{\"connectorIds\":[\"RConn1\"],\"side\":\"BOTTOM\"},\"type\":\"ConnectorPlacement.EquallySpacedRectSide\",\"uuid\":\"2353ed68-b1a1-4775-9ca9-31e268d5443b\"}]},\"type\":\"ConnectorPlacement.EquallySpacedConnector\",\"uuid\":\"d5479f4c-4e65-4791-adcb-73df11f88590\"}],\"packageUris\":[\"http://schema.mathworks.com/mf0/Connector/R2020b\"],\"version\":\"1.0\"}"
  switch_3 : Subsystem
      settings: PortSchema="{\"entries\":[{\"content\":{\"sides\":[{\"content\":{\"connectorIds\":[\"LConn1\"]},\"type\":\"ConnectorPlacement.EquallySpacedRectSide\",\"uuid\":\"9277da8d-d460-43e6-8478-dd662f15d226\"},{\"content\":{\"connectorIds\":[],\"side\":\"RIGHT\"},\"type\":\"ConnectorPlacement.EquallySpacedRectSide\",\"uuid\":\"a7ece396-f1d9-4f4f-a05b-db1fc65d6e1d\"},{\"content\":{\"connectorIds\":[\"LConn2\"],\"side\":\"TOP\"},\"type\":\"ConnectorPlacement.EquallySpacedRectSide\",\"uuid\":\"fdd70777-e9cf-4317-afb6-cae87f75d5b0\"},{\"content\":{\"connectorIds\":[\"RConn1\"],\"side\":\"BOTTOM\"},\"type\":\"ConnectorPlacement.EquallySpacedRectSide\",\"uuid\":\"2353ed68-b1a1-4775-9ca9-31e268d5443b\"}]},\"type\":\"ConnectorPlacement.EquallySpacedConnector\",\"uuid\":\"d5479f4c-4e65-4791-adcb-73df11f88590\"}],\"packageUris\":[\"http://schema.mathworks.com/mf0/Connector/R2020b\"],\"version\":\"1.0\"}"
  switch_4 : Subsystem
      settings: PortSchema="{\"entries\":[{\"content\":{\"sides\":[{\"content\":{\"connectorIds\":[\"LConn1\"]},\"type\":\"ConnectorPlacement.EquallySpacedRectSide\",\"uuid\":\"9277da8d-d460-43e6-8478-dd662f15d226\"},{\"content\":{\"connectorIds\":[],\"side\":\"RIGHT\"},\"type\":\"ConnectorPlacement.EquallySpacedRectSide\",\"uuid\":\"a7ece396-f1d9-4f4f-a05b-db1fc65d6e1d\"},{\"content\":{\"connectorIds\":[\"LConn2\"],\"side\":\"TOP\"},\"type\":\"ConnectorPlacement.EquallySpacedRectSide\",\"uuid\":\"fdd70777-e9cf-4317-afb6-cae87f75d5b0\"},{\"content\":{\"connectorIds\":[\"RConn1\"],\"side\":\"BOTTOM\"},\"type\":\"ConnectorPlacement.EquallySpacedRectSide\",\"uuid\":\"2353ed68-b1a1-4775-9ca9-31e268d5443b\"}]},\"type\":\"ConnectorPlacement.EquallySpacedConnector\",\"uuid\":\"d5479f4c-4e65-4791-adcb-73df11f88590\"}],\"packageUris\":[\"http://schema.mathworks.com/mf0/Connector/R2020b\"],\"version\":\"1.0\"}"
  uac_1(+) : PMIOPort  Side=Left
  uac_1(-) : PMIOPort  Port=2  Side=Left
  udc(+) : PMIOPort  Port=3  Side=Right
  udc(-) : PMIOPort  Port=4  Side=Right
  tag scope: ileg_dc_inv=global
  wires:
  Bus Selector/4 -> [gate_Q4]  "<gate_Q4>"
  Bus Selector/3 -> [gate_Q3]  "<gate_Q3>"
  Bus Selector/2 -> [gate_Q2]  "<gate_Q2>"
  Bus Selector/1 -> [gate_Q1]  "<gate_Q1>"
  ileg_dc_inv/1 -> [ileg_dc_inv]
  gate_commands/1 -> Bus Selector/1
  [gate_Q4] -> Simulink-PS Converter3/1
  [gate_Q3] -> Simulink-PS Converter2/1
  [gate_Q2] -> Simulink-PS Converter1/1
  [gate_Q1] -> Simulink-PS Converter/1
  connections:
  Current Sensor1/RConn1 -- ileg_dc_inv/LConn1
  switch_1/LConn2 -- Current Sensor1/RConn2
  switch_3/RConn1 -- switch_4/LConn2 -- uac_1(-)/RConn1
  switch_2/LConn2 -- switch_1/RConn1 -- uac_1(+)/RConn1
  switch_4/LConn1 -- Simulink-PS Converter3/RConn1
  switch_3/LConn1 -- Simulink-PS Converter2/RConn1
  switch_2/LConn1 -- Simulink-PS Converter1/RConn1
  switch_1/LConn1 -- Simulink-PS Converter/RConn1
  switch_2/RConn1 -- switch_4/RConn1 -- udc(-)/RConn1
  udc(+)/RConn1 -- switch_3/LConn2 -- Current Sensor1/LConn1
